simulink model "CML_Iso_Force_Matching"  (R2015a)
settings: Solver=ode4  SolverMode=MultiTasking  StartTime=0.0  StopTime=inf  FixedStep=BKIN_STEP_TIME  RelTol=1e-3
StartFcn:
  |  warndlg('Dexterit-E models cannot run under simulation. Please compile your model and run it from within Dexterit-E.');set_param(bdroot,'SimulationCommand','stop')
model workspace (MAT data in the model file):
  BKIN_STEP_TIME = 0.00025
  col_x = 1
  col_y = 2
  VRAD = 3
  COLOR = 4
  TARGET_COL = 2
  BKIN_KINEMATIC_FRAME_SIZE = 400
  E_NO_EVENT = 0
  INIT_DUR = 5
  TP_ITI = 11
  K_JOINT_ASSESSED = 3
  TEXT1 = 5
  TEXT2 = 6
  HEIGHT = 8
  STROKE_WIDTH = 9
  GOAL_F_PCT = 3
  DO_FDBK = 10
  MAX_MOVE_TIME = 9
  MIN_FORCE = 4
  E_TEST_MVC = 1
  E_HOLD_MVC = 3
  E_EOT = 30
  E_FORCE_TRIAL = 11
  E_HOLD_FORCE = 13
  K_BAR_TGT = 4
  K_MVC_TEXT_TGT = 5
  E_INIT_FORCE = 12
  E_SET_MVC = 2
  TRIAL_TYPE = 1
  TEST_ARM = 8
  E_REST_FORCE = 14
  E_INIT_MATCH_FORCE = 15
  E_HOLD_MATCH_FORCE = 16
  TEXT3 = 7
  K_MVC = 6
  E_ACCEPT_MVC = 5
  ACCEPT_MVC = 2
  REJECT_MVC = 3
  K_ARM1_TGT = 1
  K_ARM2_TGT = 2
  E_FATIGUE_TRIAL = 21
  E_INIT_FATIGUE = 22
  E_HOLD_FATIGUE = 23
  HOLD_TIME = 6
  REST_TIME = 7
  E_CHECK_MVC = 4
  E_REJECT_MVC = 6
  K_SUR_TGT = 7
  K_SUR_TEXT_TGT = 8
  TEXT4 = 10
  AUDIO_FDBK_TYPE = 12
libraries: Video x8, simulink x7, slrtlib x7, General x3, KINARM_loads x3, KINARM_IO x2, KINARM_general x2, xpcnilib x1
(part 1 of 2)
CloseFcn:
  | rtwprivate ssgencode ModelCloseRequest b2lab2d
settings Model: ModifiedComment=chris -- Wed Feb 16 09:18:30 2005 -- Version 1.1384  ExtModeArmWhenConnect=off  ExtModeLogAll=off  LastModifiedBy=User
settings SolverCC: EnableConcurrentExecution=on  AutoInsertRateTranBlk=on
settings DataIOCC: LimitDataPoints=off  SignalLoggingSaveFormat=ModelDataLogs  SaveOutput=off  SaveTime=off  SignalLoggingName=sigsOut
settings OptimizationCC: BlockReduction=off  BooleanDataType=off  OptimizeBlockIOStorage=off  BufferReuse=off  GlobalBufferReuse=off  ExpressionFolding=off  ExpressionDepthLimit=2147483647  LocalBlockOutputs=off  InitFltsAndDblsToZero=on
settings DebuggingCC: SaveWithParameterizedLinksMsg=none  UnderspecifiedInitializationDetection=Classic  MergeDetectMultiDrivingBlocksExec=none  SignalResolutionControl=TryResolveAllWithWarning  MultiTaskDSMMsg=warning  FcnCallInpInsideContextMsg=UseLocalSettings  StateNameClashWarn=warning  StrictBusMsg=ErrorOnBusTreatedAsVector
settings HardwareCC: ProdIntDivRoundTo=Zero  ProdEndianess=LittleEndian  ProdLongLongMode=on  ProdHWDeviceType=Generic->32-bit x86 compatible  TargetHWDeviceType=32-bit Generic
settings SFSimCC: SimParseCustomCode=off
settings RTWCC: SystemTargetFile=slrt.tlc  TemplateMakefile=slrt_default_tmf  Description=Simulink Real-Time  RTWCompilerOptimization=on
settings CodeAppCC: MaxIdLength=63
settings SimulinkRealTimeCC: TargetFcnLib=ansi_tfl_tmw.mat  GeneratePreprocessorConditionals=Disable all  xPCisDownloadable=off

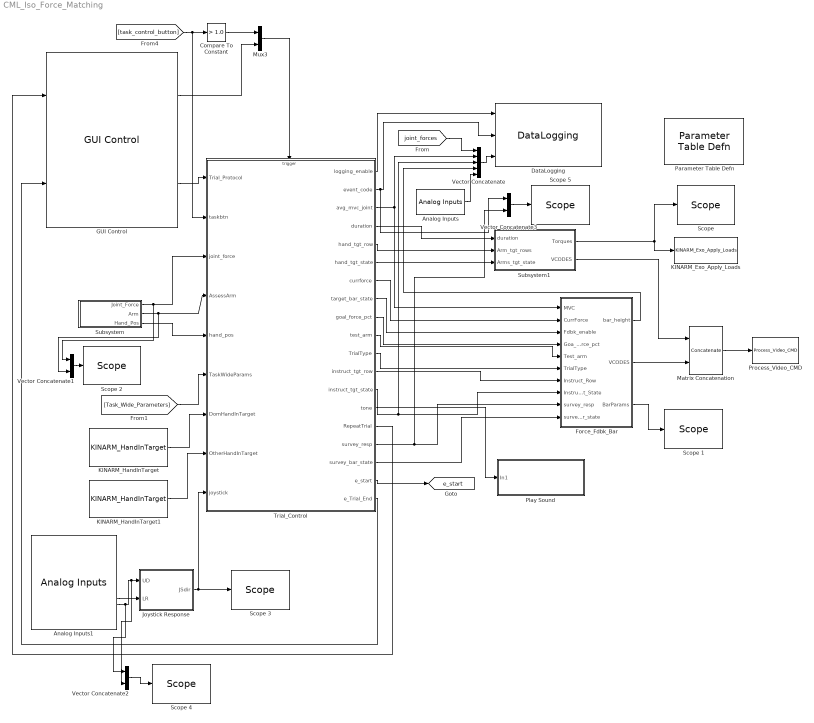
== system CML_Iso_Force_Matching ==
  Analog Inputs : KINARM_IO/Analog Inputs  channel=[1]  range=[5]  coupling=[0]  scantime6071e=1.28e-5  scantime6229=5e-6  sampletime=0.001  slot=-1  oscantime6071e=0
  Analog Inputs1 : KINARM_IO/Analog Inputs  channel=[1:32]  range=[5, 5, 5, 5, 5, 5, 5, 5,5, 5, 5, 5, 5, 5, 5, 5,5, 5, 5, 5, 5, 5, 5, 5,5, 5, 5, 5, 5, 5, 5, 5,]  coupling=[0, 0, 0, 0, 0, 0, 0, 0,0, 0, 0, 0, 0, 0, 0, 0,0, 0, 0, 0, 0, 0, 0, 0,0, 0, 0, 0, 0, 0, 0, 0,]  scantime6071e=1.28e-5  scantime6229=5e-6  sampletime=0.001  slot=-1  oscantime6071e=0
  Compare To Constant : simulink/Logic and Bit Operations/Compare To Constant  relop=>  const=1.0  OutDataTypeStr=boolean
  DataLogging : General/DataLogging  log_event_codes=on  log_analog_inputs=on  show_time_remaining=off  ecat_include=on
      link override Poll KINARM/EPTorqueCMD: GotoTag=KINARMEPTorqueCMD
      link override Poll KINARM/TorqueCMD: GotoTag=KINARMTorqueCMD
  Force_Fdbk_Bar : Subsystem
  GUI Control : General/GUI Control  task_version=1.0  show_repeat_trial_flag=on  use_custom_tp=off  target_type_str=Circle  Target_Type=1  XYcols=[1 2]  Vcols=3  Lcols=4  indices_padding=[0 0 0 0;0 0 0 0]  target_table_rows=64  load_table_rows=20  tp_table_rows=100
  Joystick Response : Subsystem
  KINARM_Exo_Apply_Loads : KINARM_loads/KINARM_Exo_Apply_Loads  up_duration=1000  down_duration=1000  max_torque=10  limit_motors=off
  KINARM_HandInTarget : KINARM_general/KINARM_HandInTarget  use_dominant_hand=on  target_type=Circle  num_states=1  attribcol1=[VRAD]  attribcol2=[0]  attribcol3=[0]  attribcol4=[0]  attribcol5=[0]
  KINARM_HandInTarget1 : KINARM_general/KINARM_HandInTarget  use_dominant_hand=off  target_type=Circle  num_states=1  attribcol1=[VRAD]  attribcol2=[0]  attribcol3=[0]  attribcol4=[0]  attribcol5=[0]
  Matrix Concatenation : Concatenate  Mode=Multidimensional array
  Mux3 : Mux  Inputs=2
  Parameter Table Defn : General/Parameter Table Defn  ShowInLibBrowser=0
  Play Sound : Subsystem
  Process_Video_CMD : Video/Process_Video_CMD  video_delay=0
  "Scope " : slrtlib/Displays and Logging/Scope   scopeno=1  scopetype=Target  autostart=on  viewmode=Numerical  formatstr='%15.6f'  grid=on  ylimits=[0,0]  nosamples=250  noprepostsamples=0  interleave=1  triggermode=FreeRun  triggersignal=1  trigsignalfromport=off  triggerlevel=0.0  triggerslope=Either  triggerscope=1  triggersample=0  filename=data.dat  mode=Lazy  writesize=512  autorestart=off  dynamicfilemode=off  maxwritefilesize=512*1024^2
  Scope 1 : slrtlib/Displays and Logging/Scope   scopeno=2  scopetype=Target  autostart=on  viewmode=Numerical  formatstr='%15.6f'  grid=on  ylimits=[0,0]  nosamples=250  noprepostsamples=0  interleave=1  triggermode=FreeRun  triggersignal=1  trigsignalfromport=off  triggerlevel=0.0  triggerslope=Either  triggerscope=1  triggersample=0  filename=data.dat  mode=Lazy  writesize=512  autorestart=off  dynamicfilemode=off  maxwritefilesize=512*1024^2
  Scope 2 : slrtlib/Displays and Logging/Scope   scopeno=3  scopetype=Target  autostart=on  viewmode=Numerical  formatstr='%15.6f'  grid=on  ylimits=[0,0]  nosamples=250  noprepostsamples=0  interleave=1  triggermode=FreeRun  triggersignal=1  trigsignalfromport=off  triggerlevel=0.0  triggerslope=Either  triggerscope=1  triggersample=0  filename=data.dat  mode=Lazy  writesize=512  autorestart=off  dynamicfilemode=off  maxwritefilesize=512*1024^2
  Scope 3 : slrtlib/Displays and Logging/Scope   scopeno=4  scopetype=Target  autostart=on  viewmode=Numerical  formatstr='%15.6f'  grid=on  ylimits=[0,0]  nosamples=250  noprepostsamples=0  interleave=1  triggermode=FreeRun  triggersignal=1  trigsignalfromport=off  triggerlevel=0.0  triggerslope=Either  triggerscope=1  triggersample=0  filename=data.dat  mode=Lazy  writesize=512  autorestart=off  dynamicfilemode=off  maxwritefilesize=512*1024^2
  Scope 4 : slrtlib/Displays and Logging/Scope   scopeno=6  scopetype=Target  autostart=on  viewmode=Numerical  formatstr='%15.6f'  grid=on  ylimits=[0,0]  nosamples=250  noprepostsamples=0  interleave=1  triggermode=FreeRun  triggersignal=1  trigsignalfromport=off  triggerlevel=0.0  triggerslope=Either  triggerscope=1  triggersample=0  filename=data.dat  mode=Lazy  writesize=512  autorestart=off  dynamicfilemode=off  maxwritefilesize=512*1024^2
  Scope 5 : slrtlib/Displays and Logging/Scope   scopeno=7  scopetype=Target  autostart=on  viewmode=Numerical  formatstr='%15.6f'  grid=on  ylimits=[0,0]  nosamples=250  noprepostsamples=0  interleave=1  triggermode=FreeRun  triggersignal=1  trigsignalfromport=off  triggerlevel=0.0  triggerslope=Either  triggerscope=1  triggersample=0  filename=data.dat  mode=Lazy  writesize=512  autorestart=off  dynamicfilemode=off  maxwritefilesize=512*1024^2
  Subsystem : Subsystem
  Subsystem1 : Subsystem
  Trial_Control : Stateflow chart  TreatAsAtomicUnit=on
  Vector Concatenate : Concatenate  NumInputs=5
  Vector Concatenate1 : Concatenate
  Vector Concatenate2 : Concatenate
  Vector Concatenate3 : Concatenate
  tag scope: e_start=global
  wires:
  Subsystem1/2(VCODES) -> Matrix Concatenation/1
  Trial_Control/19(e_Trial_End) -> GUI Control/2
  Trial_Control/6(hand_tgt_state) -> Subsystem1/3(Arms_tgt_state)
  Trial_Control/5(hand_tgt_row) -> Subsystem1/2(Arm_tgt_rows)
  Matrix Concatenation/1 -> Process_Video_CMD/1
  GUI Control/2 -> Trial_Control/1(Trial_Protocol)
  Trial_Control/1(logging_enable) -> DataLogging/1
  Subsystem1/1(Torques) -> KINARM_Exo_Apply_Loads/1, "Scope "/1
  Trial_Control/18(e_start) -> [e_start]
  [joint_forces] -> Vector Concatenate/1
  Vector Concatenate/1 -> DataLogging/3
  Analog Inputs/1 -> Vector Concatenate/5
  Subsystem/1(Joint_Force) -> Vector Concatenate1/1, Trial_Control/3(joint_force)
  Subsystem/3(Hand_Pos) -> Trial_Control/5(hand_pos)
  [Task_Wide_Parameters] -> Trial_Control/6(TaskWideParams)
  Trial_Control/12(instruct_tgt_row) -> Force_Fdbk_Bar/7(Instruct_Row)
  Trial_Control/13(instruct_tgt_state) -> Vector Concatenate/3, Force_Fdbk_Bar/8(Instruct_State)
  Trial_Control/3(avg_mvc_joint) -> Force_Fdbk_Bar/1(MVC), Vector Concatenate/2
  Force_Fdbk_Bar/2(VCODES) -> Matrix Concatenation/2
  Trial_Control/8(target_bar_state) -> Force_Fdbk_Bar/3(Fdbk_enable)
  Trial_Control/7(currforce) -> Force_Fdbk_Bar/2(CurrForce)
  Trial_Control/9(goal_force_pct) -> Force_Fdbk_Bar/4(Goa_force_pct)
  Force_Fdbk_Bar/1(bar_height) -> Vector Concatenate/4
  Force_Fdbk_Bar/3(BarParams) -> Scope 1/1
  Trial_Control/2(event_code) -> Vector Concatenate3/1, DataLogging/2
  Trial_Control/11(TrialType) -> Force_Fdbk_Bar/6(TrialType)
  KINARM_HandInTarget/1 -> Trial_Control/7(DomHandInTarget)
  Trial_Control/10(test_arm) -> Force_Fdbk_Bar/5(Test_arm)
  GUI Control/1 -> Mux3/2
  [task_control_button] -> Trial_Control/2(taskbtn), Compare To Constant/1
  Mux3/1 -> Trial_Control/Trigger
  Compare To Constant/1 -> Mux3/1
  Trial_Control/4(duration) -> Subsystem1/1(duration)
  Subsystem/2(Arm) -> Vector Concatenate1/2, Trial_Control/4(AssessArm)
  Trial_Control/14(tone) -> Play Sound/1(In1)
  Trial_Control/15(RepeatTrial) -> GUI Control/1
  KINARM_HandInTarget1/1 -> Trial_Control/8(OtherHandInTarget)
  Vector Concatenate1/1 -> Scope 2/1
  Analog Inputs1/22 -> Joystick Response/2(LR)
  Analog Inputs1/24 -> Vector Concatenate2/1, Vector Concatenate2/2, Joystick Response/1(UD)
  Joystick Response/1(JSdir) -> Scope 3/1, Trial_Control/9(joystick)
  Trial_Control/17(survey_bar_state) -> Force_Fdbk_Bar/10(survey_bar_state)
  Trial_Control/16(survey_resp) -> Vector Concatenate3/2, Force_Fdbk_Bar/9(survey_resp)
  Vector Concatenate2/1 -> Scope 4/1
  Vector Concatenate3/1 -> Scope 5/1

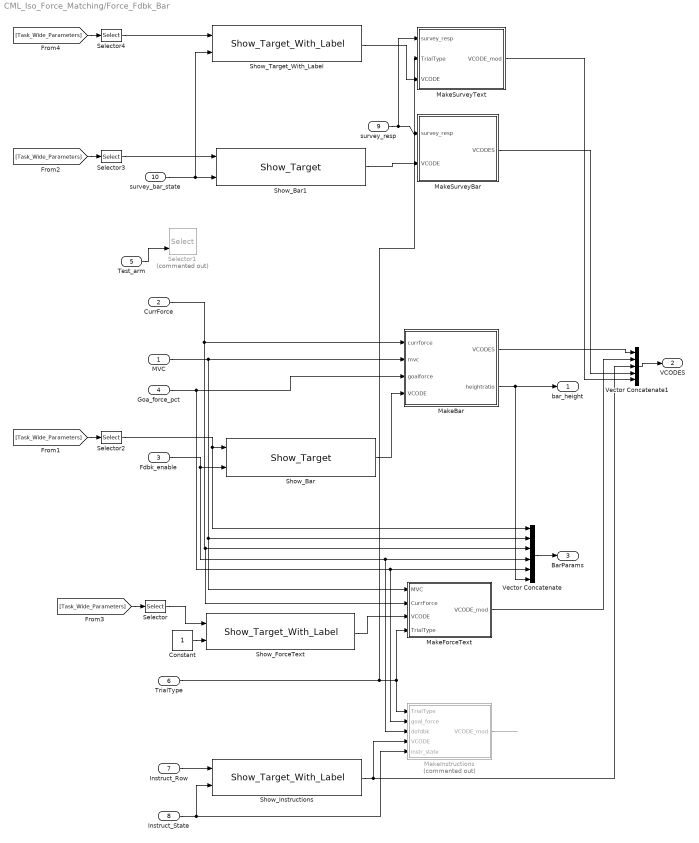
== system CML_Iso_Force_Matching/Force_Fdbk_Bar ==
  MVC : Inport
  CurrForce : Inport  Port=2
  Fdbk_enable : Inport  Port=3
  Goa_force_pct : Inport  Port=4
  Test_arm : Inport  Port=5
  TrialType : Inport  Port=6
  Instruct_Row : Inport  Port=7
  Instruct_State : Inport  Port=8
  survey_resp : Inport  Port=9
  survey_bar_state : Inport  Port=10
  Constant : Constant
  MakeBar : MATLAB Function  TreatAsAtomicUnit=on
  MakeForceText : MATLAB Function  TreatAsAtomicUnit=on
  MakeInstructions : MATLAB Function  Commented=on  TreatAsAtomicUnit=on
  MakeSurveyBar : MATLAB Function  TreatAsAtomicUnit=on
  MakeSurveyText : MATLAB Function  TreatAsAtomicUnit=on
  Selector : Selector  InputPortWidth=50  Indices=[K_MVC_TEXT_TGT]
  Selector1 : Selector  Commented=on  InputPortWidth=2  IndexOptions=Index vector (port)  Indices=[1 3]
  Selector2 : Selector  InputPortWidth=50  Indices=[K_BAR_TGT]
  Selector3 : Selector  InputPortWidth=50  Indices=[K_SUR_TGT]
  Selector4 : Selector  InputPortWidth=50  Indices=[K_SUR_TEXT_TGT]
  Show_Bar : Video/Show_Target  target_type=Rectangle  num_states=1  attribcol1=[COLOR 0 STROKE_WIDTH VRAD HEIGHT 0]  attribcol2=[0 0 0 0 0 0]  attribcol3=[0 0 0 0 0 0]  attribcol4=[0 0 0 0 0 0]  attribcol5=[0 0 0 0 0 0]  stateindices_padding=[0 0 0 0 0;0 0 0 0 0;0 0 0 0 0;0 0 0 0 0;0 0 0 0 0]  source=dialog  opacity=100  target_display=Both subject and operator displays  num_col=6
  Show_Bar1 : Video/Show_Target  target_type=Rectangle  num_states=1  attribcol1=[COLOR 0 STROKE_WIDTH VRAD HEIGHT 0]  attribcol2=[0 0 0 0 0 0]  attribcol3=[0 0 0 0 0 0]  attribcol4=[0 0 0 0 0 0]  attribcol5=[0 0 0 0 0 0]  stateindices_padding=[0 0 0 0 0;0 0 0 0 0;0 0 0 0 0;0 0 0 0 0;0 0 0 0 0]  source=dialog  opacity=100  target_display=Both subject and operator displays  num_col=6
  Show_ForceText : Video/Show_Target_With_Label  target_type=Rectangle  num_states=1  attribcol1=[0 0 0 VRAD HEIGHT 0 TEXT1 COLOR HEIGHT]  attribcol2=[0 0 0 0 0 0 0 0 0]  attribcol3=[0 0 0 0 0 0 0 0 0]  attribcol4=[0 0 0 0 0 0 0 0 0]  attribcol5=[0 0 0 0 0 0 0 0 0]  stateindices_padding=[0 0;0 0;0 0;0 0;0 0]  source=dialog  opacity=100  target_display=Operator display only
  Show_Instructions : Video/Show_Target_With_Label  target_type=Rectangle  num_states=4  attribcol1=[0 0 0 VRAD HEIGHT 0 TEXT1 COLOR HEIGHT]  attribcol2=[0 0 0 VRAD HEIGHT 0 TEXT2 COLOR HEIGHT]  attribcol3=[0 0 0 VRAD HEIGHT 0 TEXT3 COLOR HEIGHT]  attribcol4=[0 0 0 VRAD HEIGHT 0 TEXT4 COLOR HEIGHT]  attribcol5=[0 0 0 0 0 0 0 0 0]  stateindices_padding=[0 0;0 0;0 0;0 0;0 0]  source=dialog  opacity=100  target_display=Both subject and operator displays
  Show_Target_With_Label : Video/Show_Target_With_Label  target_type=Circle  num_states=1  attribcol1=[0 0 0 0 TEXT1 COLOR HEIGHT]  attribcol2=[0 0 0 0 0 0 0]  attribcol3=[0 0 0 0 0 0 0]  attribcol4=[0 0 0 0 0 0 0]  attribcol5=[0 0 0 0 0 0 0]  stateindices_padding=[0 0 0 0;0 0 0 0;0 0 0 0;0 0 0 0;0 0 0 0]  source=dialog  opacity=100  target_display=Both subject and operator displays
  Vector Concatenate : Concatenate  NumInputs=6
  Vector Concatenate1 : Concatenate  NumInputs=5  Mode=Multidimensional array
  bar_height : Outport
  VCODES : Outport  Port=2
  BarParams : Outport  Port=3
  wires:
  Fdbk_enable/1 -> MakeInstructions/3(dofdbk), Vector Concatenate/4, Show_Bar/2
  Selector2/1 -> Vector Concatenate/1, Show_Bar/1
  CurrForce/1 -> MakeBar/1(currforce), MakeForceText/2(CurrForce), Vector Concatenate/3
  MVC/1 -> MakeForceText/1(MVC), Vector Concatenate/2, MakeBar/2(mvc)
  Show_Bar/1 -> MakeBar/4(VCODE)
  MakeBar/1(VCODES) -> Vector Concatenate1/1
  Goa_force_pct/1 -> Vector Concatenate/5, MakeInstructions/2(goal_force), MakeBar/3(goalforce)
  MakeBar/2(heightratio) -> Vector Concatenate/6, bar_height/1
  Vector Concatenate/1 -> BarParams/1
  Constant/1 -> Show_ForceText/2
  Show_ForceText/1 -> MakeForceText/3(VCODE)
  MakeForceText/1(VCODE_mod) -> Vector Concatenate1/2
  Vector Concatenate1/1 -> VCODES/1
  TrialType/1 -> MakeSurveyText/2(TrialType), MakeForceText/4(TrialType), MakeInstructions/1(TrialType)
  Selector/1 -> Show_ForceText/1
  [Task_Wide_Parameters] -> Selector/1
  Instruct_Row/1 -> Show_Instructions/1
  Instruct_State/1 -> MakeInstructions/5(instr_state), Show_Instructions/2
  MakeInstructions/1(VCODE_mod) -> ?
  Test_arm/1 -> Selector1/2
  Show_Instructions/1 -> MakeInstructions/4(VCODE), Vector Concatenate1/3
  [Task_Wide_Parameters] -> Selector2/1
  survey_bar_state/1 -> Show_Target_With_Label/2, Show_Bar1/2
  [Task_Wide_Parameters] -> Selector3/1
  Selector3/1 -> Show_Bar1/1
  Show_Bar1/1 -> MakeSurveyBar/2(VCODE)
  survey_resp/1 -> MakeSurveyText/1(survey_resp), MakeSurveyBar/1(survey_resp)
  MakeSurveyBar/1(VCODES) -> Vector Concatenate1/4
  [Task_Wide_Parameters] -> Selector4/1
  Selector4/1 -> Show_Target_With_Label/1
  Show_Target_With_Label/1 -> MakeSurveyText/3(VCODE)
  MakeSurveyText/1(VCODE_mod) -> Vector Concatenate1/5

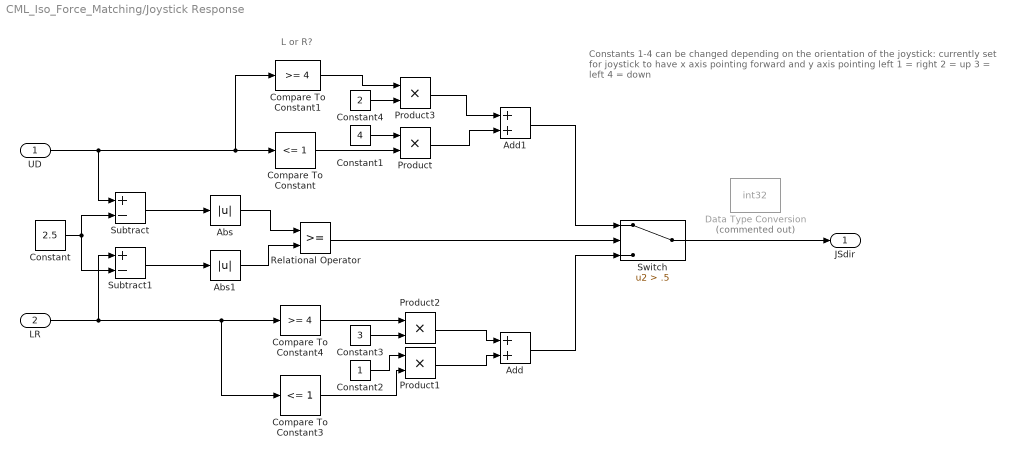
== system CML_Iso_Force_Matching/Joystick Response ==
  note: Constants 1-4 can be changed depending on the orientation of the joystick:
      | currently set for joystick to have x axis pointing forward and y axis pointing left
      |
      | 1 = right
      | 2 = up
      | 3 = left
      | 4 = down
  note: L or R?
  UD : Inport
  LR : Inport  Port=2
  Abs : Abs
  Abs1 : Abs
  Add : Sum
  Add1 : Sum
  Compare To Constant : simulink/Logic and Bit Operations/Compare To Constant  relop=<=  const=1  OutDataTypeStr=boolean
  Compare To Constant1 : simulink/Logic and Bit Operations/Compare To Constant  relop=>=  const=4  OutDataTypeStr=boolean
  Compare To Constant3 : simulink/Logic and Bit Operations/Compare To Constant  relop=<=  const=1  OutDataTypeStr=boolean
  Compare To Constant4 : simulink/Logic and Bit Operations/Compare To Constant  relop=>=  const=4  OutDataTypeStr=boolean
  Constant : Constant  Value=2.5
  Constant1 : Constant  Value=4
  Constant2 : Constant
  Constant3 : Constant  Value=3
  Constant4 : Constant  Value=2
  Data Type Conversion : DataTypeConversion  Commented=on  OutDataTypeStr=int32
  Product{,1..3} (4 alike) : Product
  Relational Operator : RelationalOperator  OutDataTypeStr=boolean
  Subtract : Sum  Inputs=+-
  Subtract1 : Sum  Inputs=+-
  Switch : Switch  Criteria=u2 > Threshold  Threshold=.5
  JSdir : Outport
  wires:
  UD/1 -> Compare To Constant1/1, Compare To Constant/1, Subtract/1
  Compare To Constant/1 -> Product/2
  LR/1 -> Compare To Constant3/1, Compare To Constant4/1, Subtract1/1
  Compare To Constant3/1 -> Product1/2
  Compare To Constant4/1 -> Product2/1
  Subtract/1 -> Abs/1
  Subtract1/1 -> Abs1/1
  Constant/1 -> Subtract/2, Subtract1/2
  Abs/1 -> Relational Operator/1
  Abs1/1 -> Relational Operator/2
  Compare To Constant1/1 -> Product3/1
  Constant1/1 -> Product/1
  Constant2/1 -> Product1/1
  Constant3/1 -> Product2/2
  Product2/1 -> Add/1
  Product1/1 -> Add/2
  Product/1 -> Add1/2
  Add1/1 -> Switch/1
  Add/1 -> Switch/3
  Relational Operator/1 -> Switch/2
  Constant4/1 -> Product3/2
  Product3/1 -> Add1/1
  Switch/1 -> JSdir/1

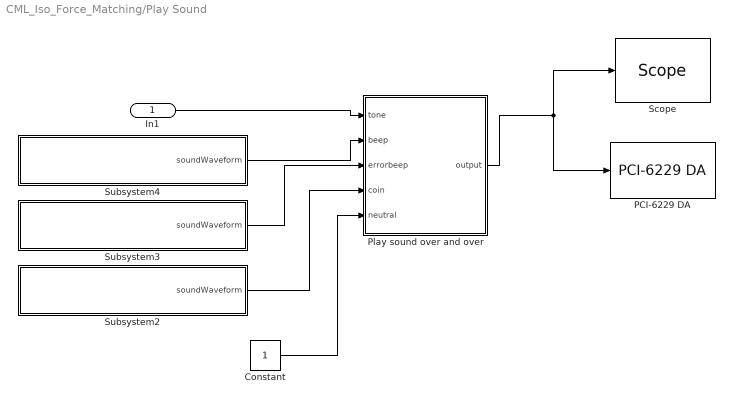
== system CML_Iso_Force_Matching/Play Sound ==
  In1 : Inport
  Constant : Constant
  PCI-6229 DA : xpcnilib/D//A/M Series/PCI-6229 DA  channel=[1]  reset=[1]  initValue=[0]  sampletime=-1  slot=-1
  Play sound over and over : MATLAB Function  TreatAsAtomicUnit=on
  "Scope " : slrtlib/Displays and Logging/Scope   scopeno=5  scopetype=Target  autostart=on  viewmode=Graphical redraw  formatstr='%15.6f'  grid=on  ylimits=[0,0]  nosamples=4000  noprepostsamples=0  interleave=1  triggermode=FreeRun  triggersignal=1  trigsignalfromport=off  triggerlevel=0.0  triggerslope=Either  triggerscope=1  triggersample=0  filename=data.dat  mode=Lazy  writesize=512  autorestart=off  dynamicfilemode=off  maxwritefilesize=512*1024^2
  Subsystem2 : Subsystem  mask(Load Waveform Into Variable){fileName=coin.mat}
      mask prompts: fileName "Name of .mat Data File (must be in current directory)"
      mask help: This block will load the .MAT file specified in the dialog, and put the first variable into a GoTo called 'soundWaveform'.
      mask init:
      | filenameFromMask = get_param(gcb, 'fileName');
      | 
      | try 
      | 	dataFromFile = load(filenameFromMask);
      | 	names = fieldnames(dataFromFile);
      | 	soundDataFromFile = dataFromFile.(names{1});
      | 	display(['Sound waveform from file ''' filenameFromMask ''' loaded.']);
      | catch ME
      | 	display(ME.message)
      | end
      mask Help:
      | Enter the name a .MAT file containing a single vector or matrix. The .MAT file must be located in the current directory.
      | 
      | The first variable from the .MAT file will be put into a Goto called 'soundWaveform'.
      mask Display: disp(['Load waveform from ''' filenameFromMask ''''])
  Subsystem3 : Subsystem  mask(Load Waveform Into Variable){fileName=errorbeep.mat}
      mask prompts: fileName "Name of .mat Data File (must be in current directory)"
      mask help: This block will load the .MAT file specified in the dialog, and put the first variable into a GoTo called 'soundWaveform'.
      mask init: same as CML_Iso_Force_Matching/Play Sound/Subsystem2
      mask Help:
      | Enter the name a .MAT file containing a single vector or matrix. The .MAT file must be located in the current directory.
      | 
      | The first variable from the .MAT file will be put into a Goto called 'soundWaveform'.
      mask Display: disp(['Load waveform from ''' filenameFromMask ''''])
  Subsystem4 : Subsystem  mask(Load Waveform Into Variable){fileName=startbeep.mat}
      mask prompts: fileName "Name of .mat Data File (must be in current directory)"
      mask help: This block will load the .MAT file specified in the dialog, and put the first variable into a GoTo called 'soundWaveform'.
      mask init: same as CML_Iso_Force_Matching/Play Sound/Subsystem2
      mask Help:
      | Enter the name a .MAT file containing a single vector or matrix. The .MAT file must be located in the current directory.
      | 
      | The first variable from the .MAT file will be put into a Goto called 'soundWaveform'.
      mask Display: disp(['Load waveform from ''' filenameFromMask ''''])
  wires:
  Play sound over and over/1(output) -> PCI-6229 DA/1, "Scope "/1
  Subsystem3/1(soundWaveform) -> Play sound over and over/3(errorbeep)
  Subsystem4/1(soundWaveform) -> Play sound over and over/2(beep)
  In1/1 -> Play sound over and over/1(tone)
  Subsystem2/1(soundWaveform) -> Play sound over and over/4(coin)
  Constant/1 -> Play sound over and over/5(neutral)

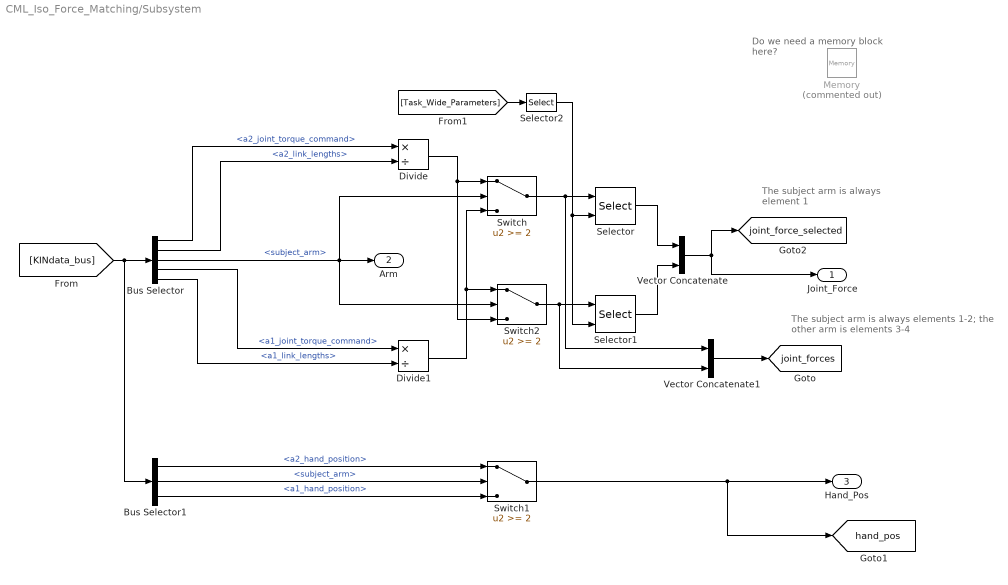
== system CML_Iso_Force_Matching/Subsystem ==
  note: Do we need a memory block here?
  note: The subject arm is always element 1
  note: The subject arm is always elements 1-2; the other arm is elements 3-4
  Bus Selector : BusSelector  OutputSignals=Robot2.a2_joint_torque_command,Robot2.a2_link_lengths,KINDataGeneral.subject_arm,Robot1.a1_joint_torque_command,Robot1.a1_link_lengths
  Bus Selector1 : BusSelector  OutputSignals=Robot2.a2_hand_position,KINDataGeneral.subject_arm,Robot1.a1_hand_position
  Divide : Product  Inputs=*/
  Divide1 : Product  Inputs=*/
  Memory : Memory  Commented=on
  Selector : Selector  InputPortWidth=2  IndexOptions=Index vector (port)  Indices=[1 3]
  Selector1 : Selector  InputPortWidth=2  IndexOptions=Index vector (port)  Indices=[1 3]
  Selector2 : Selector  InputPortWidth=50  Indices=[K_JOINT_ASSESSED]
  Switch : Switch  Threshold=2
  Switch1 : Switch  Threshold=2
  Switch2 : Switch  Threshold=2
  Vector Concatenate : Concatenate
  Vector Concatenate1 : Concatenate
  Joint_Force : Outport
  Arm : Outport  Port=2
  Hand_Pos : Outport  Port=3
  tag scope: hand_pos=global, joint_force_selected=global, joint_forces=global
  wires:
  [KINdata_bus] -> Bus Selector1/1, Bus Selector/1
  Bus Selector/3 -> Arm/1, Switch/2, Switch2/2  "<subject_arm>"
  Divide/1 -> Switch2/3, Switch/1
  Divide1/1 -> Switch2/1, Switch/3
  Bus Selector/1 -> Divide/1  "<a2_joint_torque_command>"
  Bus Selector/2 -> Divide/2  "<a2_link_lengths>"
  Bus Selector/4 -> Divide1/1  "<a1_joint_torque_command>"
  Bus Selector/5 -> Divide1/2  "<a1_link_lengths>"
  Bus Selector1/1 -> Switch1/1  "<a2_hand_position>"
  Bus Selector1/2 -> Switch1/2  "<subject_arm>"
  Bus Selector1/3 -> Switch1/3  "<a1_hand_position>"
  Switch/1 -> Selector/1, Vector Concatenate1/1
  Selector2/1 -> Selector1/2, Selector/2
  Switch1/1 -> [hand_pos], Hand_Pos/1
  Vector Concatenate/1 -> [joint_force_selected], Joint_Force/1
  Switch2/1 -> Selector1/1, Vector Concatenate1/2
  Selector/1 -> Vector Concatenate/1
  Selector1/1 -> Vector Concatenate/2
  Vector Concatenate1/1 -> [joint_forces]
  [Task_Wide_Parameters] -> Selector2/1

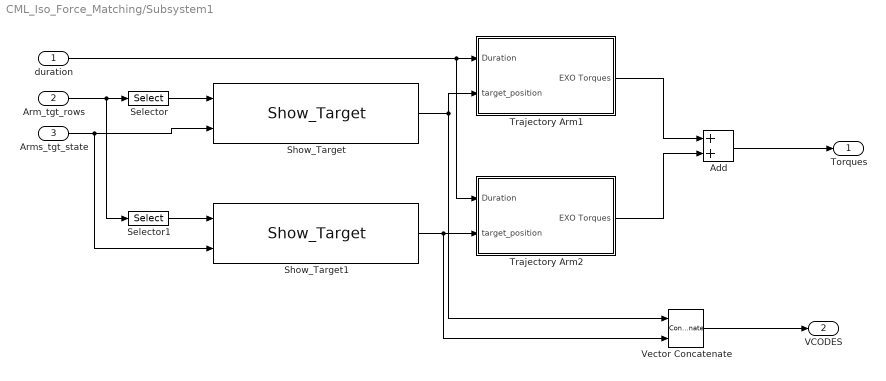
== system CML_Iso_Force_Matching/Subsystem1 ==
  duration : Inport
  Arm_tgt_rows : Inport  Port=2
  Arms_tgt_state : Inport  Port=3
  Add : Sum
  Selector : Selector  InputPortWidth=2  Indices=[1]
  Selector1 : Selector  InputPortWidth=2  Indices=[2]
  Show_Target : Video/Show_Target  target_type=Circle  num_states=1  attribcol1=[COLOR 0 0 VRAD]  attribcol2=[0 0 0 0]  attribcol3=[0 0 0 0]  attribcol4=[0 0 0 0]  attribcol5=[0 0 0 0]  stateindices_padding=[0 0 0 0 0 0 0;0 0 0 0 0 0 0;0 0 0 0 0 0 0;0 0 0 0 0 0 0;0 0 0 0 0 0 0]  source=dialog  opacity=100  target_display=Both subject and operator displays  num_col=4
  Show_Target1 : Video/Show_Target  target_type=Circle  num_states=1  attribcol1=[COLOR 0 0 VRAD]  attribcol2=[0 0 0 0]  attribcol3=[0 0 0 0]  attribcol4=[0 0 0 0]  attribcol5=[0 0 0 0]  stateindices_padding=[0 0 0 0 0 0 0;0 0 0 0 0 0 0;0 0 0 0 0 0 0;0 0 0 0 0 0 0;0 0 0 0 0 0 0]  source=dialog  opacity=100  target_display=Both subject and operator displays  num_col=4
  Trajectory Arm1 : Subsystem
  Trajectory Arm2 : Subsystem
  Vector Concatenate : Concatenate  Mode=Multidimensional array
  Torques : Outport
  VCODES : Outport  Port=2
  wires:
  Show_Target/1 -> Trajectory Arm1/2(target_position), Vector Concatenate/1
  duration/1 -> Trajectory Arm2/1(Duration), Trajectory Arm1/1(Duration)
  Arm_tgt_rows/1 -> Selector/1, Selector1/1
  Arms_tgt_state/1 -> Show_Target1/2, Show_Target/2
  Show_Target1/1 -> Vector Concatenate/2, Trajectory Arm2/2(target_position)
  Trajectory Arm1/1(EXO Torques) -> Add/1
  Trajectory Arm2/1(EXO Torques) -> Add/2
  Add/1 -> Torques/1
  Selector/1 -> Show_Target/1
  Selector1/1 -> Show_Target1/1
  Vector Concatenate/1 -> VCODES/1

== system CML_Iso_Force_Matching/Play Sound/Subsystem2 ==
  Constant1 : Constant  Value=soundDataFromFile
  soundWaveform : Outport
  wires:
  Constant1/1 -> soundWaveform/1

== system CML_Iso_Force_Matching/Play Sound/Subsystem3 ==
  Constant1 : Constant  Value=soundDataFromFile
  soundWaveform : Outport
  wires:
  Constant1/1 -> soundWaveform/1

== system CML_Iso_Force_Matching/Play Sound/Subsystem4 ==
  Constant1 : Constant  Value=soundDataFromFile
  soundWaveform : Outport
  wires:
  Constant1/1 -> soundWaveform/1

== system CML_Iso_Force_Matching/Subsystem1/Trajectory Arm1 ==
  note: In the Position Controller dialog, the "Time base of desired Position input signal" was set to 0.001.
      | This value is different from the Simulink sample-time of 0.0005 for that signal because the calculations
      | that create that signal in the Create_Trajectory block are based on 1 kHz. Please see the Help for
      | Position Controller block for more details.
  Duration : Inport
  target_position : Inport  Port=2
  Create_Trajectory : Subsystem
  KINARM_Exo_Position_Controller : KINARM_loads/KINARM_Exo_Position_Controller  use_dom_hand=on  KINARM_Type=Human  inertias_for_FF=KINARM robot & arm troughs  angles_or_XY=End-point (global x/y)  sample_time=0.001
  calculate robot scaling : Subsystem
  EXO Torques : Outport
  wires:
  Create_Trajectory/2(reset_controller) -> KINARM_Exo_Position_Controller/2
  Create_Trajectory/1(virtual_position) -> KINARM_Exo_Position_Controller/1
  KINARM_Exo_Position_Controller/1 -> EXO Torques/1
  target_position/1 -> Create_Trajectory/3(target_position)
  Duration/1 -> Create_Trajectory/1(nominal_duration)
  [e_start] -> Create_Trajectory/2(e_start)
  calculate robot scaling/1(scaling) -> Create_Trajectory/4(robot scaling)

== system CML_Iso_Force_Matching/Subsystem1/Trajectory Arm2 ==
  note: In the Position Controller dialog, the "Time base of desired Position input signal" was set to 0.001.
      | This value is different from the Simulink sample-time of 0.0005 for that signal because the calculations
      | that create that signal in the Create_Trajectory block are based on 1 kHz. Please see the Help for
      | Position Controller block for more details.
  Duration : Inport
  target_position : Inport  Port=2
  Create_Trajectory : Subsystem
  KINARM_Exo_Position_Controller : KINARM_loads/KINARM_Exo_Position_Controller  use_dom_hand=off  KINARM_Type=Human  inertias_for_FF=KINARM robot & arm troughs  angles_or_XY=End-point (global x/y)  sample_time=0.001
  calculate robot scaling : Subsystem
  EXO Torques : Outport
  wires:
  Create_Trajectory/2(reset_controller) -> KINARM_Exo_Position_Controller/2
  Create_Trajectory/1(virtual_position) -> KINARM_Exo_Position_Controller/1
  KINARM_Exo_Position_Controller/1 -> EXO Torques/1
  target_position/1 -> Create_Trajectory/3(target_position)
  Duration/1 -> Create_Trajectory/1(nominal_duration)
  [e_start] -> Create_Trajectory/2(e_start)
  calculate robot scaling/1(scaling) -> Create_Trajectory/4(robot scaling)

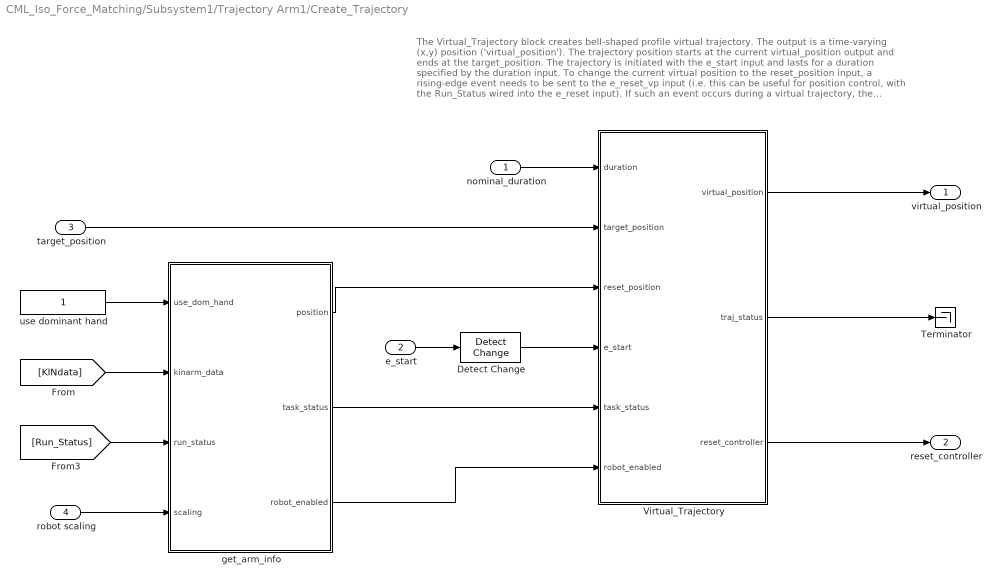
== system CML_Iso_Force_Matching/Subsystem1/Trajectory Arm1/Create_Trajectory ==
  note: The Virtual_Trajectory block creates bell-shaped profile virtual trajectory.
      | The output is a time-varying (x,y) position ('virtual_position').
      |
      | The trajectory position starts at the current virtual_position output and ends at the target_position.
      | The trajectory is initiated with the e_start input and lasts for a duration specified by the duration input.
      |
      | To change the current virtual position to the reset_position input, a rising-edge event needs to be sent to the e_reset_vp input
      | (i.e. this can be useful for position control, with the Run_Status wired into the e_reset input).
      | If such an event occurs during a virtual trajectory, the trajectory is halted immediately.
  nominal_duration : Inport
  e_start : Inport  Port=2
  target_position : Inport  Port=3
  robot scaling : Inport  Port=4
  Detect Change : simulink/Logic and Bit Operations/Detect Change  vinit=0  InputProcessing=Inherited  OutDataTypeStr=uint8
  Terminator : Terminator
  Virtual_Trajectory : Subsystem
  get_arm_info : MATLAB Function  TreatAsAtomicUnit=on
  use dominant hand : Constant
  virtual_position : Outport
  reset_controller : Outport  Port=2
  wires:
  Virtual_Trajectory/1(virtual_position) -> virtual_position/1
  nominal_duration/1 -> Virtual_Trajectory/1(duration)
  e_start/1 -> Detect Change/1
  target_position/1 -> Virtual_Trajectory/2(target_position)
  Detect Change/1 -> Virtual_Trajectory/4(e_start)
  use dominant hand/1 -> get_arm_info/1(use_dom_hand)
  [KINdata] -> get_arm_info/2(kinarm_data)
  get_arm_info/1(position) -> Virtual_Trajectory/3(reset_position)
  Virtual_Trajectory/3(reset_controller) -> reset_controller/1
  get_arm_info/2(task_status) -> Virtual_Trajectory/5(task_status)
  get_arm_info/3(robot_enabled) -> Virtual_Trajectory/6(robot_enabled)
  [Run_Status] -> get_arm_info/3(run_status)
  Virtual_Trajectory/2(traj_status) -> Terminator/1
  robot scaling/1 -> get_arm_info/4(scaling)

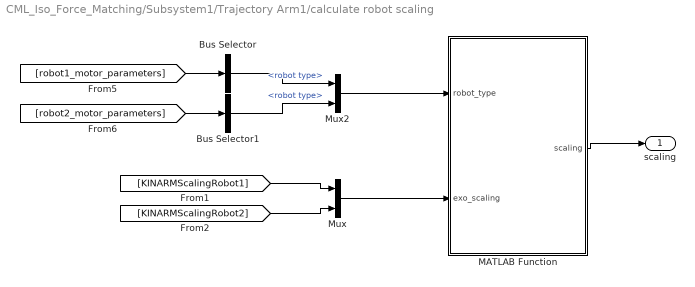
== system CML_Iso_Force_Matching/Subsystem1/Trajectory Arm1/calculate robot scaling ==
  Bus Selector : BusSelector  OutputSignals=robot type
  Bus Selector1 : BusSelector  OutputSignals=robot type
  MATLAB Function : MATLAB Function  TreatAsAtomicUnit=on
  Mux : Mux  Inputs=2
  Mux2 : Mux  Inputs=2
  scaling : Outport
  wires:
  [KINARMScalingRobot1] -> Mux/1
  [KINARMScalingRobot2] -> Mux/2
  Mux/1 -> MATLAB Function/2(exo_scaling)
  Mux2/1 -> MATLAB Function/1(robot_type)
  MATLAB Function/1(scaling) -> scaling/1
  [robot2_motor_parameters] -> Bus Selector1/1
  Bus Selector1/1 -> Mux2/2  "<robot type>"
  Bus Selector/1 -> Mux2/1  "<robot type>"
  [robot1_motor_parameters] -> Bus Selector/1

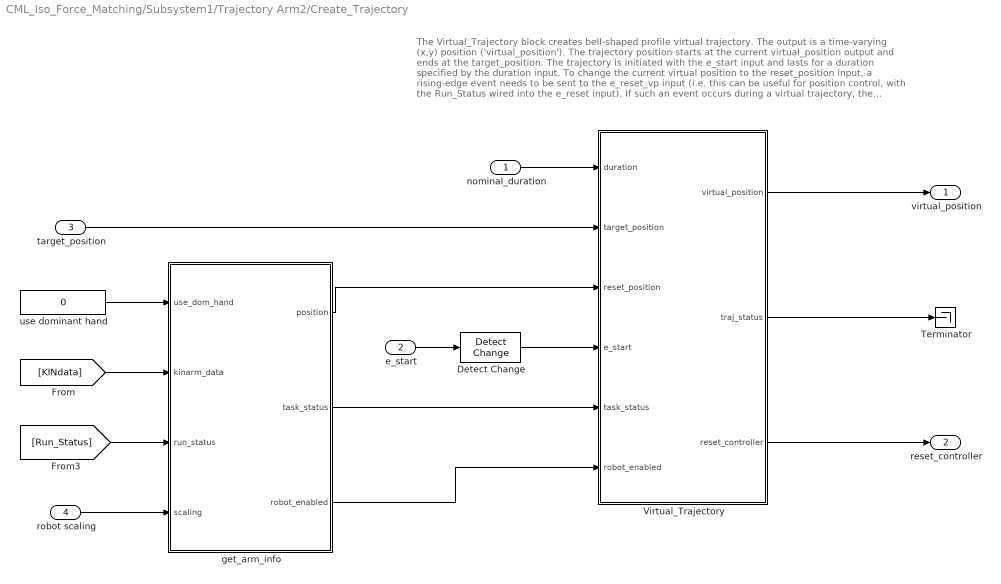
== system CML_Iso_Force_Matching/Subsystem1/Trajectory Arm2/Create_Trajectory ==
  note: The Virtual_Trajectory block creates bell-shaped profile virtual trajectory.
      | The output is a time-varying (x,y) position ('virtual_position').
      |
      | The trajectory position starts at the current virtual_position output and ends at the target_position.
      | The trajectory is initiated with the e_start input and lasts for a duration specified by the duration input.
      |
      | To change the current virtual position to the reset_position input, a rising-edge event needs to be sent to the e_reset_vp input
      | (i.e. this can be useful for position control, with the Run_Status wired into the e_reset input).
      | If such an event occurs during a virtual trajectory, the trajectory is halted immediately.
  nominal_duration : Inport
  e_start : Inport  Port=2
  target_position : Inport  Port=3
  robot scaling : Inport  Port=4
  Detect Change : simulink/Logic and Bit Operations/Detect Change  vinit=0  InputProcessing=Inherited  OutDataTypeStr=uint8
  Terminator : Terminator
  Virtual_Trajectory : Subsystem
  get_arm_info : MATLAB Function  TreatAsAtomicUnit=on
  use dominant hand : Constant  Value=0
  virtual_position : Outport
  reset_controller : Outport  Port=2
  wires:
  Virtual_Trajectory/1(virtual_position) -> virtual_position/1
  nominal_duration/1 -> Virtual_Trajectory/1(duration)
  e_start/1 -> Detect Change/1
  target_position/1 -> Virtual_Trajectory/2(target_position)
  Detect Change/1 -> Virtual_Trajectory/4(e_start)
  use dominant hand/1 -> get_arm_info/1(use_dom_hand)
  [KINdata] -> get_arm_info/2(kinarm_data)
  get_arm_info/1(position) -> Virtual_Trajectory/3(reset_position)
  Virtual_Trajectory/3(reset_controller) -> reset_controller/1
  get_arm_info/2(task_status) -> Virtual_Trajectory/5(task_status)
  get_arm_info/3(robot_enabled) -> Virtual_Trajectory/6(robot_enabled)
  [Run_Status] -> get_arm_info/3(run_status)
  Virtual_Trajectory/2(traj_status) -> Terminator/1
  robot scaling/1 -> get_arm_info/4(scaling)

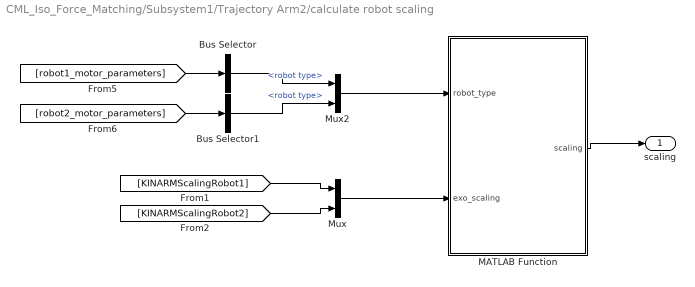
== system CML_Iso_Force_Matching/Subsystem1/Trajectory Arm2/calculate robot scaling ==
  Bus Selector : BusSelector  OutputSignals=robot type
  Bus Selector1 : BusSelector  OutputSignals=robot type
  MATLAB Function : MATLAB Function  TreatAsAtomicUnit=on
  Mux : Mux  Inputs=2
  Mux2 : Mux  Inputs=2
  scaling : Outport
  wires:
  [KINARMScalingRobot1] -> Mux/1
  [KINARMScalingRobot2] -> Mux/2
  Mux/1 -> MATLAB Function/2(exo_scaling)
  Mux2/1 -> MATLAB Function/1(robot_type)
  MATLAB Function/1(scaling) -> scaling/1
  [robot2_motor_parameters] -> Bus Selector1/1
  Bus Selector1/1 -> Mux2/2  "<robot type>"
  Bus Selector/1 -> Mux2/1  "<robot type>"
  [robot1_motor_parameters] -> Bus Selector/1

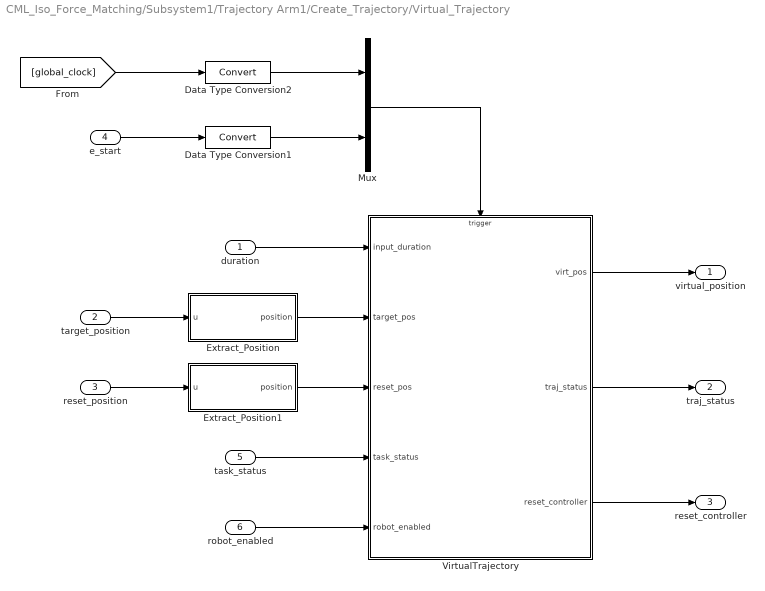
== system CML_Iso_Force_Matching/Subsystem1/Trajectory Arm1/Create_Trajectory/Virtual_Trajectory ==
  duration : Inport
  target_position : Inport  Port=2
  reset_position : Inport  Port=3
  e_start : Inport  Port=4
  task_status : Inport  Port=5
  robot_enabled : Inport  Port=6
  Data Type Conversion1 : DataTypeConversion
  Data Type Conversion2 : DataTypeConversion
  Extract_Position : MATLAB Function  TreatAsAtomicUnit=on
  Extract_Position1 : MATLAB Function  TreatAsAtomicUnit=on
  Mux : Mux  Inputs=2
  VirtualTrajectory : Stateflow chart  TreatAsAtomicUnit=on
  virtual_position : Outport
  traj_status : Outport  Port=2
  reset_controller : Outport  Port=3
  wires:
  e_start/1 -> Data Type Conversion1/1
  target_position/1 -> Extract_Position/1(u)
  [global_clock] -> Data Type Conversion2/1
  Mux/1 -> VirtualTrajectory/Trigger
  duration/1 -> VirtualTrajectory/1(input_duration)
  VirtualTrajectory/1(virt_pos) -> virtual_position/1
  Extract_Position/1(position) -> VirtualTrajectory/2(target_pos)
  reset_position/1 -> Extract_Position1/1(u)
  Data Type Conversion2/1 -> Mux/1
  VirtualTrajectory/2(traj_status) -> traj_status/1
  robot_enabled/1 -> VirtualTrajectory/5(robot_enabled)
  task_status/1 -> VirtualTrajectory/4(task_status)
  Data Type Conversion1/1 -> Mux/2
  Extract_Position1/1(position) -> VirtualTrajectory/3(reset_pos)
  VirtualTrajectory/3(reset_controller) -> reset_controller/1

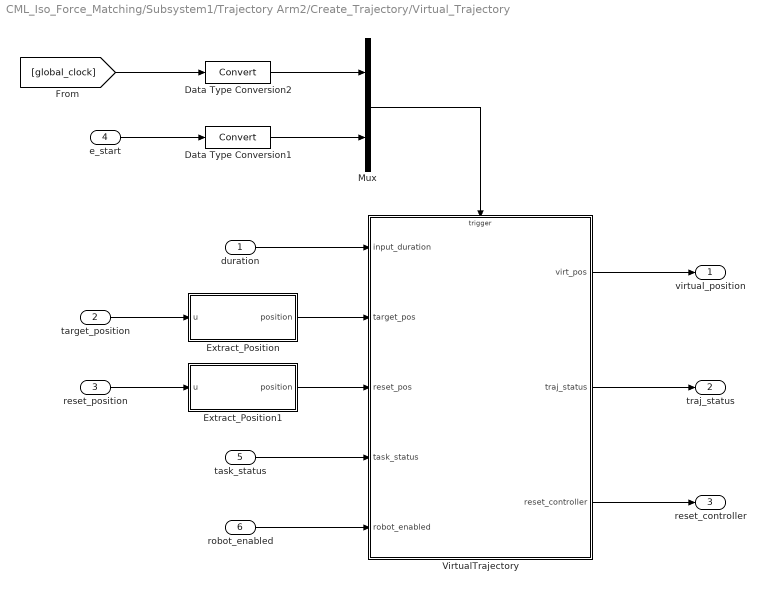
== system CML_Iso_Force_Matching/Subsystem1/Trajectory Arm2/Create_Trajectory/Virtual_Trajectory ==
  duration : Inport
  target_position : Inport  Port=2
  reset_position : Inport  Port=3
  e_start : Inport  Port=4
  task_status : Inport  Port=5
  robot_enabled : Inport  Port=6
  Data Type Conversion1 : DataTypeConversion
  Data Type Conversion2 : DataTypeConversion
  Extract_Position : MATLAB Function  TreatAsAtomicUnit=on
  Extract_Position1 : MATLAB Function  TreatAsAtomicUnit=on
  Mux : Mux  Inputs=2
  VirtualTrajectory : Stateflow chart  TreatAsAtomicUnit=on
  virtual_position : Outport
  traj_status : Outport  Port=2
  reset_controller : Outport  Port=3
  wires:
  e_start/1 -> Data Type Conversion1/1
  target_position/1 -> Extract_Position/1(u)
  [global_clock] -> Data Type Conversion2/1
  Mux/1 -> VirtualTrajectory/Trigger
  duration/1 -> VirtualTrajectory/1(input_duration)
  VirtualTrajectory/1(virt_pos) -> virtual_position/1
  Extract_Position/1(position) -> VirtualTrajectory/2(target_pos)
  reset_position/1 -> Extract_Position1/1(u)
  Data Type Conversion2/1 -> Mux/1
  VirtualTrajectory/2(traj_status) -> traj_status/1
  robot_enabled/1 -> VirtualTrajectory/5(robot_enabled)
  task_status/1 -> VirtualTrajectory/4(task_status)
  Data Type Conversion1/1 -> Mux/2
  Extract_Position1/1(position) -> VirtualTrajectory/3(reset_pos)
  VirtualTrajectory/3(reset_controller) -> reset_controller/1

== stateflow chart CML_Iso_Force_Matching/Trial_Control ==
  settings: sampleTime=0.001
  state init/
    //bring the hand to the start position
    mvc_joint = 0;
    n_mvc = 1*(avg_mvc_joint > 1e-4);
    avg_mvc_joint = TaskWideParams[K_MVC];
    hand_tgt_row[1] = TaskWideParams[K_ARM1_TGT];
    hand_tgt_row[2] = TaskWideParams[K_ARM2_TGT];
    hand_tgt_state = 1;
    test_arm = 1; //1 means subject assessment arm, 2 means opposite arm
    instruct_tgt_row = 0;
    instruct_tgt_state = 0;
    duration = 3000;
  state Main_Trial
    state InitFatigueTrial/
      event_code = E_FATIGUE_TRIAL;
      logging_enable = 1;
      duration = 1;
      instruct_tgt_row = Trial_Protocol[TARGET_COL];
      instruct_tgt_state = 1;
      tmpforce = 0;
      tmpcounter = 0;
      iforce = 0;
      maxforce = 0;
      goal_force_pct = Trial_Protocol[GOAL_F_PCT];
      goal_force = avg_mvc_joint*(goal_force_pct/100.0);
      target_bar_state = Trial_Protocol[DO_FDBK];
      min_force = Trial_Protocol[MIN_FORCE];
      force_thresh = min_force;
      force_thresh += force_thresh*(target_bar_state == 0); //if no feedback, relax the criterion
      test_arm = Trial_Protocol[TEST_ARM];
      hold_time = Trial_Protocol[HOLD_TIME];
      max_move_time = Trial_Protocol[MAX_MOVE_TIME];
      tick = 0;
      tone = 1;
    state InitSurveyTrial/
      // Init the survey and parameters
      // Just needs to update, display happens in VCODE section
      event_code = E_SURVEY_INIT;
      logging_enable = 1;
      instruct_tgt_row = Trial_Protocol[TARGET_COL];
      instruct_tgt_state = 4;
      survey_bar_state=1;
      survey_resp=4;
      survey_delta = 1;
    state InitForceTrial/
      event_code = E_FORCE_TRIAL;
      logging_enable = 1;
      duration = 1;
      instruct_tgt_row = Trial_Protocol[TARGET_COL];
      instruct_tgt_state = 1;
      tmpforce = 0;
      tmpcounter = 0;
      iforce = 0;
      maxforce = 0;
      goal_force_pct = Trial_Protocol[GOAL_F_PCT];
      goal_force = avg_mvc_joint*(goal_force_pct/100.0);
      target_bar_state = Trial_Protocol[DO_FDBK];
      min_force = Trial_Protocol[MIN_FORCE];
      force_thresh = min_force;
      force_thresh += force_thresh*(target_bar_state == 0); //if no feedback, relax the criterion
      test_arm = 1;
      hold_time = Trial_Protocol[HOLD_TIME];
      max_move_time = Trial_Protocol[MAX_MOVE_TIME];
      tick = 0;
      tone = 1;
      during:
      currforce = joint_force[1];
    state InitMVC/
      event_code = E_TEST_MVC;
      logging_enable = 1;
      duration = 1;
      instruct_tgt_row = Trial_Protocol[TARGET_COL];
      instruct_tgt_state = 1;
      target_bar_state = 0;
      min_force = Trial_Protocol[MIN_FORCE];
      tmpforce = 0;
      maxforce = min_force;
      currforce = 0;
      test_arm = 1;
      hold_time = Trial_Protocol[HOLD_TIME];
      max_move_time = Trial_Protocol[MAX_MOVE_TIME];
      tick = 0;
      tone = 1;
    state SurveyIncrease/
      event_code=E_SURVEY_INC;
      survey_resp+=survey_delta;
    state SurveyMain/
      // Main block, set termination conditioin later
      // All options loop back to this block
      event_code=E_SURVEY_MAIN;
      during:
      response=joystick;
    state SurveyDecrease/
      event_code=E_SURVEY_DEC;
      survey_resp-=survey_delta;
    state FatigueApplyForce/
      event_code = E_INIT_FATIGUE;
      during:
      maxforce = joint_force[test_arm];
      currforce = joint_force[test_arm];
      tmpcounter = 0;
      tick++;
    state ApplyForce/
      event_code = E_INIT_FORCE;
      during:
      maxforce = joint_force[1];
      tmpcounter = 0;
      tick++;
      currforce = joint_force[1];
    state SetMVC/
      event_code = E_SET_MVC;
      tmpcounter = 0;
      tmp_forcehist = 0;
      iforce = 0;
      during: //check and update the estimated mvc
      tick++;
      currforce = joint_force[1];
      [maxforce,iforce, tmp_forcehist] = calcmvc(tmp_forcehist,iforce,currforce)
    state HoldMVC/
      event_code = E_HOLD_MVC;
      tone = 0;
      during: //check and update the estimated mvc
      tick++;
      tmpcounter++;
      currforce = joint_force[1];
    state HoldFatigueForce/
      event_code = E_HOLD_FATIGUE;
      tone = 0;
      instruct_tgt_state = 3;
      during:
      maxforce = joint_force[test_arm];
      currforce = joint_force[test_arm];
      tmpcounter++;
      tick++;
    state HoldAppliedForce/
      event_code = E_HOLD_FORCE;
      tone = 0;
      during:
      maxforce = joint_force[1];
      currforce = joint_force[1];
      tmpcounter++;
      tick++;
    state WaitAcceptMVC/
      event_code = E_CHECK_MVC;
      currforce = maxforce;
      instruct_tgt_state = 2;
      tone = 1;
    state Ready/
      instruct_tgt_state = 3;
      test_arm = Trial_Protocol[TEST_ARM];
      tick = 0;
      tmpcounter = 0;
      tone = 1;
      during:
      currforce = joint_force[test_arm];
    state Rest1/
      instruct_tgt_state = 2;
      target_bar_state = 0;
      during:
      currforce = joint_force[1];
    state Rest2/
      event_code = E_REST_FORCE;
      duration = Trial_Protocol[REST_TIME];
    state AcceptMVC/
      event_code = E_ACCEPT_MVC;
      //record the MVC on this trial if desired
      mvc_joint += maxforce; %*(tmpcounter >= force_hold_time);
      n_mvc += 1; %*(tmpcounter >= force_hold_time);
      avg_mvc_joint = mvc_joint/n_mvc;
    state EndOfFatigueTrial/
      event_code = E_EOT;
      instruct_tgt_state = 2;
      TrialType = 0;
      tone = 2;
    state EndOfTrial1/
      event_code = E_EOT;
      instruct_tgt_state = 2;
      survey_bar_state=0;
      TrialType = 0;
    state EndMVC/
      event_code = E_EOT;
      instruct_tgt_state = 2;
    state ApplyForce2/
      event_code = E_INIT_MATCH_FORCE;
      during:
      maxforce = joint_force[test_arm];
      currforce = joint_force[test_arm];
      tmpcounter = 0;
      tick++;
    state HoldAppliedForce2/
      event_code = E_HOLD_MATCH_FORCE;
      during:
      maxforce = joint_force[test_arm];
      currforce = joint_force[test_arm];
      tmpcounter++;
      tick++;
    state EndOfTrial/
      event_code = E_EOT;
      instruct_tgt_state = 2;
      TrialType = 0;
    (junction 75) -> InitFatigueTrial [order 1] : [TrialType == 3]
    (junction 75) -> InitMVC [order 3] : [TrialType == 1]
    (junction 75) -> InitForceTrial [order 2] : [TrialType == 2]/
    EndOfTrial -> InitSurveyTrial : [joint_force[test_arm] <= min_force]
    InitSurveyTrial -> SurveyMain : after(1,e_clk)
    SurveyMain -> SurveyIncrease [order 1] : [response==2 && survey_resp<8]
    SurveyIncrease -> (junction 213) : after(1,e_clk)
    (junction 213) -> SurveyMain : [after(500,e_clk)]/
        | response=0;
    SurveyDecrease -> (junction 213) : after(1,e_clk)
    SurveyMain -> EndOfTrial1 [order 3] : [after(4000,e_clk)]
    SurveyMain -> SurveyDecrease [order 2] : [response == 4 && survey_resp>0]
    InitFatigueTrial -> FatigueApplyForce : [(joint_force[test_arm] > min_force) && after(1, e_clk)]
    InitForceTrial -> ApplyForce : [(joint_force[1] > min_force) && after(1, e_clk)]
    InitMVC -> SetMVC : [(joint_force[1] > min_force) && after(1, e_clk)]
    FatigueApplyForce -> EndOfFatigueTrial [order 1] : [(tick > max_move_time) ]
    SetMVC -> HoldMVC [order 1] : [abs(joint_force[1] - maxforce) < min_force]
    FatigueApplyForce -> HoldFatigueForce [order 2] : [joint_force[test_arm] > goal_force]
    HoldFatigueForce -> FatigueApplyForce [order 1] : [abs(joint_force[test_arm] - goal_force) > force_thresh]/
        | //apply the force threshold on either side of the goal
    ApplyForce -> HoldAppliedForce : [joint_force[1] > goal_force]
    HoldAppliedForce -> ApplyForce [order 1] : [abs(joint_force[1] - goal_force) > force_thresh]/
        | //apply the force threshold on either side of the goal
    HoldMVC -> SetMVC [order 2] : [abs(joint_force[1]-maxforce) > min_force]
    HoldMVC -> WaitAcceptMVC [order 1] : [(tmpcounter >= hold_time)]
    SetMVC -> WaitAcceptMVC [order 2] : [(tick > max_move_time) ]
    HoldAppliedForce -> Rest1 [order 2] : [(tmpcounter > hold_time) || (tick > max_move_time) ]
    HoldFatigueForce -> EndOfFatigueTrial [order 2] : [(tmpcounter > hold_time) || (tick > max_move_time) ]
    WaitAcceptMVC -> AcceptMVC [order 1] : [taskbtn == 2]
    Rest2 -> Ready : after(duration,e_clk)
    WaitAcceptMVC -> EndMVC [order 2] : [taskbtn == 3]/
        | RepeatTrial = 1;
        | event_code = E_REJECT_MVC;
    Rest1 -> Rest2 : [joint_force[1] < min_force]
    Ready -> ApplyForce2 : [(joint_force[test_arm] > min_force) && after(1, e_clk)]
    EndOfFatigueTrial -> (junction 111) : [joint_force[1] <= min_force]
    AcceptMVC -> EndMVC
    EndOfTrial1 -> (junction 111) : after(1,e_clk)
    ApplyForce2 -> EndOfTrial [order 1] : [(tick > max_move_time) ]/
        | tone = 3;
    EndMVC -> (junction 111) : [joint_force[1] <= min_force]
    ApplyForce2 -> HoldAppliedForce2 [order 2] : [abs(joint_force[test_arm] - goal_force) < force_thresh]
        | //see if we get close to the matching goal
    HoldAppliedForce2 -> ApplyForce2 [order 1] : [abs(joint_force[test_arm] - goal_force) > force_thresh]/
        | //apply the force threshold on either side of the goal
    HoldAppliedForce2 -> EndOfTrial [order 2] : [(tmpcounter > hold_time) || (tick > max_move_time) ]/
        | tone = 2;
  state MovToStart/
    ITI = Trial_Protocol[TP_ITI];
    TrialType = Trial_Protocol[TRIAL_TYPE];
    e_start;
    tone = 0;
  state Inter_Trial_State/
    e_Trial_End
    duration = Trial_Protocol[INIT_DUR];
  state WaitForFlagToSet
  state MeasureMVC1/ [commented out]
    event_code = E_HOLD_MVC;
    during: //check and update the estimated mvc
    [tmpforce, tmpcounter, iforce, maxforce] = update_mvc(tmpforce,joint_force,tmpcounter, iforce, maxforce, min_force);
    tick++;
  (default) -> init
  init -> (junction 85)
  (junction 85) -> MovToStart
  MovToStart -> (junction 75) : [after(duration, e_clk) && DomHandInTarget[hand_tgt_row[1]] && OtherHandInTarget[hand_tgt_row[2]] ]/
      | hand_tgt_state = 0;
  Inter_Trial_State -> (junction 85)
  WaitForFlagToSet -> Inter_Trial_State : after(2, e_clk)
  Main_Trial -> WaitForFlagToSet : e_ExitTrialNow/
      | instruct_tgt_state = 0;
      | hand_tgt_state = 0;
      | logging_enable = 0;
      | tickCount = 10;
  (junction 111) -> Inter_Trial_State : after(ITI, e_clk)
  data: forcehist function_input double size=[200,1]; itrial function_input double; meanmvc function_output double; itrial1 function_output double; force function_input double; forcehist1 function_output double size=[200,1]; currMVC function_input double; currForce function_input double; newMVC function_output double; newcount function_output double; currcount function_input double; imvc function_input double; imvc1 function_output double; max_mvc function_input double; newmax_mvc function_output double; minforce function_input double; logging_enable output boolean; event_code output double; avg_mvc_joint output double; mvc_joint local double; duration output double; hand_tgt_row output size=2 [1..32]; hand_tgt_state output double; currforce output double; tickCount local double; Trial_Protocol input double; taskbtn input double; max_move_time local double size=1; joint_force input double size=2; AssessArm input double; target_bar_state output double; goal_force_pct output double; test_arm output double; TrialType output double; hand_pos input double size=2; TaskWideParams input double size=50; instruct_tgt_row output double; instruct_tgt_state output double; n_mvc local double; tmp_forcehist local double size=[200,1] =0; tmp_counter local double; iforce local double; hold_time local double; goal_force local double; maxforce local double; min_force local double; tick local double; tmpcounter local double; tmpforce local double; ITI local double; DomHandInTarget input double; force_thresh local double; tone output double; RepeatTrial output double; OtherHandInTarget input double; joystick input double; survey_resp output double; survey_bar_state output double; response local double; survey_delta local double
  data hand_tgt_row settings: description=index of the row currently being used in the TargetTable
  data joint_force settings: description=index 1 is the assessment arm; index 2 is the opposite arm
  events: e_btn input RISING_EDGE_EVENT; e_start output EITHER_EDGE_EVENT; e_clk input RISING_EDGE_EVENT; e_ExitTrialNow input EITHER_EDGE_EVENT; e_Trial_End output EITHER_EDGE_EVENT
  function [meanmvc,itrial1, forcehist1] = calcmvc(forcehist,itrial,force):
    | function [meanmvc,itrial1, forcehist1] = calcmvc(forcehist,itrial,force)
    |  
    |  
    | itrial1 = itrial+1;
    | if itrial1 > length(forcehist)
    |     itrial1 = 1;
    | end
    | 
    | forcehist(itrial1) = force;
    | 
    | meanmvc = sum(forcehist)/sum(forcehist > 0);
    | 
    | forcehist1 = forcehist;
    | 
    | 
    | %meanmvc = mean(nonzeros(forcehist));
  function [newMVC,newcount, imvc1, newmax_mvc] = update_mvc(currMVC,currForce, currcount, imvc, max_mvc, minforce):
    | function [newMVC,newcount, imvc1, newmax_mvc] = update_mvc(currMVC,currForce, currcount, imvc, max_mvc, minforce)
    | 
    | meanmvc = mean(currMVC);
    | newMVC = currMVC;
    | 
    | forcethresh = minforce;
    | 
    | %keep a running history of applied forces
    | imvc1 = imvc+1;
    | if imvc1 > length(newMVC)
    |     imvc1 = 1;
    | end
    | 
    | newMVC(imvc1) = currForce;
    | 
    | if (currForce-meanmvc) > forcethresh  %current force is greater than the current average recorded force
    |     newcount = 0;
    |     newmax_mvc = meanmvc;
    | elseif abs(currForce-meanmvc) < forcethresh %current force is within range of current average recorded force
    |     newcount = currcount+1;
    |     newmax_mvc = meanmvc;
    | else %current force is less than range of current average recorded force
    |     newcount = 0;
    |     newmax_mvc = max_mvc;
    | end
